simulink model "TestFilter"  (Simulink 6.6)
settings: Solver=ode45  StartTime=0.0  StopTime=10.0  RelTol=1e-3
undefined symbols (not defined in the file or in its folder): DiscIntNeverNeededParam, floatToBytes, gaind, polesd, u1, y1, zerosd
libraries: simulink x22, dsPICdrivers x15, aerolibguid x1, aerolibutil x1, dspmtrx3 x1
(part 2 of 2)

== system TestFilter/Position-Attitude Filter/Position/Attitude Filter/Position  Complementary Filter/3vector LPF/Low Pass2 ==
  In1 : Inport
  Discrete Zero-Pole : DiscreteZeroPole  Zeros=zerosd  Poles=polesd  Gain=gaind  SampleTime=SampleTime
  Out1 : Outport
  wires:
  Discrete Zero-Pole/1 -> Out1/1
  In1/1 -> Discrete Zero-Pole/1

== system TestFilter/Position-Attitude Filter/Position/Attitude Filter/Position  Complementary Filter/3vector LPF/Low Pass3 ==
  In1 : Inport
  Discrete Zero-Pole : DiscreteZeroPole  Zeros=zerosd  Poles=polesd  Gain=gaind  SampleTime=SampleTime
  Out1 : Outport
  wires:
  In1/1 -> Discrete Zero-Pole/1
  Discrete Zero-Pole/1 -> Out1/1

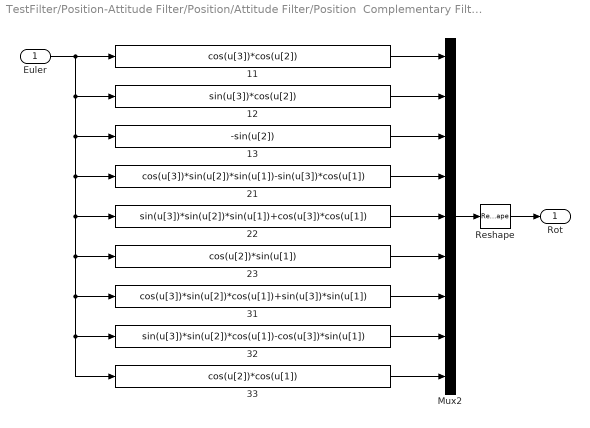
== system TestFilter/Position-Attitude Filter/Position/Attitude Filter/Position  Complementary Filter/Subsystem/RB2LTP ==
  Euler : Inport
  11 : Fcn  Expr=cos(u[3])*cos(u[2])
  12 : Fcn  Expr=sin(u[3])*cos(u[2])
  13 : Fcn  Expr=-sin(u[2])
  21 : Fcn  Expr=cos(u[3])*sin(u[2])*sin(u[1])-sin(u[3])*cos(u[1])
  22 : Fcn  Expr=sin(u[3])*sin(u[2])*sin(u[1])+cos(u[3])*cos(u[1])
  23 : Fcn  Expr=cos(u[2])*sin(u[1])
  31 : Fcn  Expr=cos(u[3])*sin(u[2])*cos(u[1])+sin(u[3])*sin(u[1])
  32 : Fcn  Expr=sin(u[3])*sin(u[2])*cos(u[1])-cos(u[3])*sin(u[1])
  33 : Fcn  Expr=cos(u[2])*cos(u[1])
  Mux2 : Mux  Inputs=9
  Reshape : Reshape  OutputDimensionality=Customize  OutputDimensions=[3,3]
  Rot : Outport
  wires:
  Reshape/1 -> Rot/1
  Euler/1 -> 12/1, 13/1, 21/1, 22/1, 23/1, 31/1, 32/1, 33/1, 11/1
  Mux2/1 -> Reshape/1
  11/1 -> Mux2/1
  12/1 -> Mux2/2
  13/1 -> Mux2/3
  21/1 -> Mux2/4
  22/1 -> Mux2/5
  23/1 -> Mux2/6
  31/1 -> Mux2/7
  32/1 -> Mux2/8
  33/1 -> Mux2/9

== system TestFilter/Position-Attitude Filter/Position/Attitude Filter/Attitude Complementary Filter/Compute Euler/Get COG/Greater than or equal to zero ==
  In1 : Inport
  Enable : EnablePort
  Out1 : Outport
  wires:
  In1/1 -> Out1/1

== system TestFilter/Position-Attitude Filter/Position/Attitude Filter/Attitude Complementary Filter/Compute Euler/Get COG/less than zero ==
  In1 : Inport
  Enable : EnablePort
  Constant : Constant  Value=2*pi  OutDataTypeMode=single
  Sum : Sum  Inputs=|++
  Out1 : Outport
  wires:
  Sum/1 -> Out1/1
  In1/1 -> Sum/1
  Constant/1 -> Sum/2

== system TestFilter/Position-Attitude Filter/Position/Attitude Filter/Attitude Complementary Filter/Compute Euler/get Centripetal/3vector LPF ==
  In1 : Inport  Orientation=left
  Demux : Demux  Orientation=left  Outputs=3
  Low Pass1 : Subsystem  Orientation=left  mask(DiscretizedZeroPole){Zeros=[], Poles=[-flpf], Gain=flpf, AbsTol=auto, SampleTime=T, method=tustin, Wc=1}
      mask prompts: Zeros "Zeros (enter in s-main:)"; Poles "Poles (enter in s-domain:)"; Gain "Gain (enter in s-domain:)"; AbsTol "Absolute tolerance:"; SampleTime "Sample time:"; Wc "Critical Frequency (Hz):"
      mask help: Continuous mask uses c2d to transform parameters onto the Discrete Zero-Pole block inside.
      mask init: same as TestFilter/Position-Attitude Filter/Position/Attitude Filter/Attitude Complementary Filter/3vector LPF/Low Pass1
      mask StyleString: edit,edit,edit,edit,edit,popup(zoh|foh|tustin|prewarp|matched),edit
      mask CallbackString: |||||hidecrit|
      mask Display:
      | droots(zeross,poless,gainss)
      | text( 0.5, 1.0, method, 'verticalAlignment','top')
  Low Pass2 : Subsystem  Orientation=left  mask(DiscretizedZeroPole){Zeros=[], Poles=[-flpf], Gain=flpf, AbsTol=auto, SampleTime=T, method=tustin, Wc=1}
      mask prompts: Zeros "Zeros (enter in s-main:)"; Poles "Poles (enter in s-domain:)"; Gain "Gain (enter in s-domain:)"; AbsTol "Absolute tolerance:"; SampleTime "Sample time:"; Wc "Critical Frequency (Hz):"
      mask help: Continuous mask uses c2d to transform parameters onto the Discrete Zero-Pole block inside.
      mask init: same as TestFilter/Position-Attitude Filter/Position/Attitude Filter/Attitude Complementary Filter/3vector LPF/Low Pass1
      mask StyleString: edit,edit,edit,edit,edit,popup(zoh|foh|tustin|prewarp|matched),edit
      mask CallbackString: |||||hidecrit|
      mask Display:
      | droots(zeross,poless,gainss)
      | text( 0.5, 1.0, method, 'verticalAlignment','top')
  Low Pass3 : Subsystem  Orientation=left  mask(DiscretizedZeroPole){Zeros=[], Poles=[-flpf], Gain=flpf, AbsTol=auto, SampleTime=T, method=tustin, Wc=1}
      mask prompts: Zeros "Zeros (enter in s-main:)"; Poles "Poles (enter in s-domain:)"; Gain "Gain (enter in s-domain:)"; AbsTol "Absolute tolerance:"; SampleTime "Sample time:"; Wc "Critical Frequency (Hz):"
      mask help: Continuous mask uses c2d to transform parameters onto the Discrete Zero-Pole block inside.
      mask init: same as TestFilter/Position-Attitude Filter/Position/Attitude Filter/Attitude Complementary Filter/3vector LPF/Low Pass1
      mask StyleString: edit,edit,edit,edit,edit,popup(zoh|foh|tustin|prewarp|matched),edit
      mask CallbackString: |||||hidecrit|
      mask Display:
      | droots(zeross,poless,gainss)
      | text( 0.5, 1.0, method, 'verticalAlignment','top')
  Mux : Mux  Orientation=left  Inputs=3
  Out1 : Outport  Orientation=left
  wires:
  Demux/1 -> Low Pass1/1(In1)
  Demux/2 -> Low Pass2/1(In1)
  Demux/3 -> Low Pass3/1(In1)
  Low Pass1/1(Out1) -> Mux/1
  Low Pass2/1(Out1) -> Mux/2
  Low Pass3/1(Out1) -> Mux/3
  In1/1 -> Demux/1
  Mux/1 -> Out1/1

== system TestFilter/Position-Attitude Filter/Position/Attitude Filter/Attitude Complementary Filter/Compute Euler/get Centripetal/3vector LPF/Low Pass1 ==
  In1 : Inport
  Discrete Zero-Pole : DiscreteZeroPole  Zeros=zerosd  Poles=polesd  Gain=gaind  SampleTime=SampleTime
  Out1 : Outport
  wires:
  In1/1 -> Discrete Zero-Pole/1
  Discrete Zero-Pole/1 -> Out1/1

== system TestFilter/Position-Attitude Filter/Position/Attitude Filter/Attitude Complementary Filter/Compute Euler/get Centripetal/3vector LPF/Low Pass2 ==
  In1 : Inport
  Discrete Zero-Pole : DiscreteZeroPole  Zeros=zerosd  Poles=polesd  Gain=gaind  SampleTime=SampleTime
  Out1 : Outport
  wires:
  Discrete Zero-Pole/1 -> Out1/1
  In1/1 -> Discrete Zero-Pole/1

== system TestFilter/Position-Attitude Filter/Position/Attitude Filter/Attitude Complementary Filter/Compute Euler/get Centripetal/3vector LPF/Low Pass3 ==
  In1 : Inport
  Discrete Zero-Pole : DiscreteZeroPole  Zeros=zerosd  Poles=polesd  Gain=gaind  SampleTime=SampleTime
  Out1 : Outport
  wires:
  In1/1 -> Discrete Zero-Pole/1
  Discrete Zero-Pole/1 -> Out1/1

== matlab function Position-Attitude Filter/Position/Attitude Filter/Attitude Complementary Filter/Compute Euler/myMux Fun ==
  data: u1 input inherited; y output inherited; u2 input inherited
function y = myMux(u1, u2)
% This block supports an embeddable subset of the MATLAB language.
% See the help menu for details. 

y = zeros(3,1);
y(1) = u1(1);
y(2) = u1(2);
y(3) = u2(1);

== matlab function Position-Attitude Filter/Position/Attitude Filter/Attitude Complementary Filter/Compute Euler/Get Roll, Pitch/myMux Fun ==
  data: u1 input inherited; y output inherited; u2 input inherited
function y = myMux(u1, u2)
% This block supports an embeddable subset of the MATLAB language.
% See the help menu for details. 

y = zeros(2,1);
y(1) = u1(1);
y(2) = u2(1);

== matlab function Position-Attitude Filter/Position/Attitude Filter/Attitude Complementary Filter/Embedded MATLAB Function1 ==
  data: euler input inherited; pqr input inherited; euler_dot output inherited
function euler_dot = Q(euler, pqr)
% This block supports an embeddable subset of the MATLAB language.
% See the help menu for details. 
p = pqr(1);
q = pqr(2);
r = pqr(3);
ph = euler(1);
th = euler(2);


euler_dot = zeros(3,1);
euler_dot(1) = p + (q*sin(ph) + r*cos(ph))*tan(th);
euler_dot(2) = q*cos(ph) - r*sin(ph);
euler_dot(3) = (q*sin(ph) + r*cos(ph))/cos(th);

== matlab function Position-Attitude Filter/Position/Attitude Filter/Attitude Complementary Filter/Embedded MATLAB Function ==
  data: euler input inherited; pqr input inherited; euler_dot output inherited
function euler_dot = Q(euler, pqr)
% This block supports an embeddable subset of the MATLAB language.
% See the help menu for details. 
p = pqr(1);
q = pqr(2);
r = pqr(3);
ph = euler(1);
th = euler(2);


euler_dot = zeros(3,1);
euler_dot(1) = p + (q*sin(ph) + r*cos(ph))*tan(th);
euler_dot(2) = q*cos(ph) - r*sin(ph);
euler_dot(3) = (q*sin(ph) + r*cos(ph))/cos(th);

== matlab function Position-Attitude Filter/Position/Attitude Filter/Attitude Complementary Filter/inertial to body ==
  data: euler input inherited; pqr output inherited; euler_dot input inherited
function pqr = Q_inv(euler,euler_dot)

phi   = euler(1);
theta = euler(2);

pqr = zeros(3,1);

pqr(1) = euler_dot(1)                   -sin(theta)*euler_dot(3);
pqr(2) =         cos(phi)*euler_dot(2)  +cos(theta)*sin(phi)*euler_dot(3);
pqr(3) =        -sin(phi)*euler_dot(2)  +cos(theta)*cos(phi)*euler_dot(3);

== matlab function Position-Attitude Filter/Position/Attitude Filter/Attitude Complementary Filter/branch cuts ==
  data: euler_in input inherited size=3; euler_out output inherited
function euler_out   = fcn(euler_in)

euler_out=zeros(3,1);

%euler_out(1)=mod(euler_in(1)+pi,2*pi)-pi;
euler_out(1)=euler_in(1);
euler_out(2)=euler_in(2);
euler_out(3)=mod(euler_in(3)+pi,2*pi)-pi;

== matlab function Position-Attitude Filter/Position/Attitude Filter/Attitude Complementary Filter/branch cuts1 ==
  data: euler_in input inherited size=3; euler_out output inherited
function euler_out   = fcn(euler_in)

euler_out=zeros(3,1);

%euler_out(1)=mod(euler_in(1)+pi,2*pi)-pi;
euler_out(1)=euler_in(1);
euler_out(2)=euler_in(2);
euler_out(3)=mod(euler_in(3),2*pi);
